simulink model "MAT_Function"  (R2020a)
settings: Solver=FixedStepAuto  StartTime=0.0  StopTime=10.0  FixedStep=1  RelTol=1e-3
libraries: simulink x2
settings Model: Creator=ashok  LastModifiedBy=ashok
settings DataIOCC: ExternalInput=[t, u,v]  LoadExternalInput=on

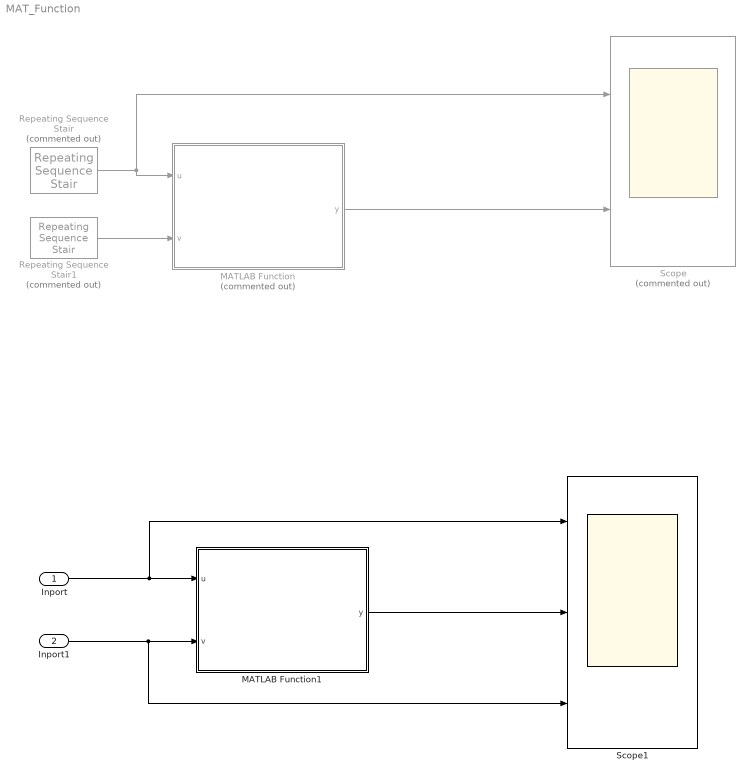
== system MAT_Function ==
  Inport : Inport
  Inport1 : Inport  Port=2
  MATLAB Function : MATLAB Function  Commented=on  TreatAsAtomicUnit=on
  MATLAB Function1 : MATLAB Function  TreatAsAtomicUnit=on
  Repeating Sequence Stair : simulink/Sources/Repeating Sequence Stair  Commented=on  OutValues=[1 -5 4 0 2.5].'  tsamp=-1  OutMin=[]  OutMax=[]  OutDataTypeStr=double  OutputDataTypeScalingMode=double  OutDataType=fixdt(0,8)  ConRadixGroup=Best Precision: Vector-wise  OutScaling=2^-12
  Repeating Sequence Stair1 : simulink/Sources/Repeating Sequence Stair  Commented=on  OutValues=[1 -5 4 0 2.5].'  tsamp=-1  OutMin=[]  OutMax=[]  OutDataTypeStr=double  OutputDataTypeScalingMode=double  OutDataType=fixdt(0,8)  ConRadixGroup=Best Precision: Vector-wise  OutScaling=2^-12
  Scope : Scope  Commented=on  NumInputPorts=2
  Scope1 : Scope  NumInputPorts=3
  wires:
  Repeating Sequence Stair/1 -> MATLAB Function/1(u), Scope/1
  MATLAB Function/1(y) -> Scope/2
  Repeating Sequence Stair1/1 -> MATLAB Function/2(v)
  Inport/1 -> Scope1/1, MATLAB Function1/1(u)
  Inport1/1 -> Scope1/3, MATLAB Function1/2(v)
  MATLAB Function1/1(y) -> Scope1/2

== matlab function MAT_Function/MATLAB Function ==
  data: u input; y output; v input
function y  = fcn(u,v)
%#codegen

if (u > 2.5)
    y = 1;
elseif ((u >= 0) && (u <= 2.5))
    y = 0;
else
    y = -1;
end

== matlab function MAT_Function/MATLAB Function1 ==
  data: u input; y output; v input
function y  = fcn(u,v)
%#codegen

if ((u >= 10) && (v >= 20))
    y = 2;
elseif ((u >= 10) && (v <= 20))
    y = 1;
else
    y = 0;
end
